simulink model "autopilot"  (R2016b)
settings: Solver=VariableStepAuto  StartTime=0.0  StopTime=sim_time  RelTol=1e-3
values from neighbouring files (symbols this model uses):
  d = 0    [run_task_2e.m]
  k_i_chi = omega_n_chi^2 * V_g / g    [prob2b.m]
  k_p_chi = 2 * zeta_chi * omega_n_chi * V_g / g    [prob2b.m]
undefined symbols (not defined in the file or in its folder): a_phi_1, a_phi_2, delta_a_max, g, k_d_phi, k_i_phi, k_p_phi, V_g
libraries: aerolibconvert2 x1
settings Model: Creator=Alexandra  LastModifiedBy=HenningWard

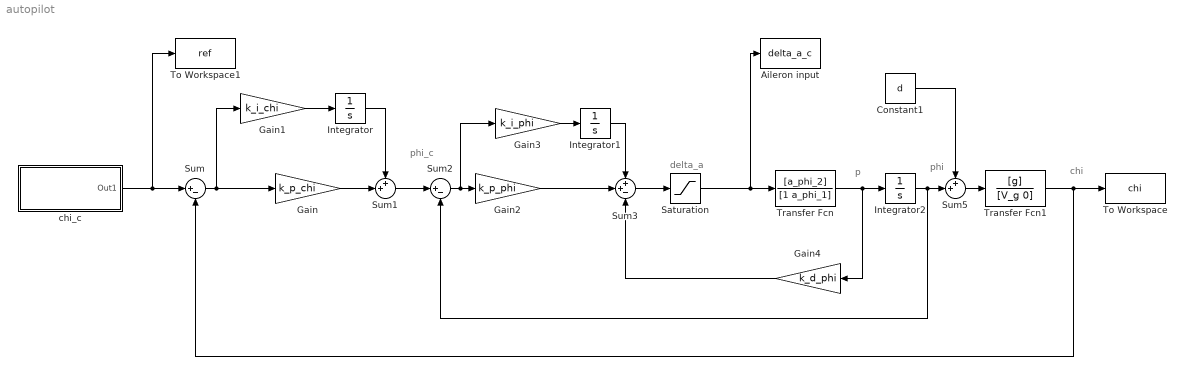
== system autopilot ==
  note: phi_c
  note: delta_a
  note: phi
  note: chi
  note: p
  Aileron input : ToWorkspace  VariableName=delta_a_c  SaveFormat=Structure With Time  SampleTime=-1
  Constant1 : Constant  Value=d
  Gain : Gain  Gain=k_p_chi
  Gain1 : Gain  Gain=k_i_chi
  Gain2 : Gain  Gain=k_p_phi
  Gain3 : Gain  Gain=k_i_phi
  Gain4 : Gain  Gain=k_d_phi
  Integrator : Integrator
  Integrator1 : Integrator
  Integrator2 : Integrator
  Saturation : Saturate  UpperLimit=delta_a_max  LowerLimit=-delta_a_max
  Sum : Sum  Inputs=|+-
  Sum1 : Sum  Inputs=++|
  Sum2 : Sum  Inputs=|+-
  Sum3 : Sum  Inputs=++-
  Sum5 : Sum  Inputs=++|
  To Workspace : ToWorkspace  VariableName=chi  SaveFormat=Structure With Time  SampleTime=-1
  To Workspace1 : ToWorkspace  VariableName=ref  SaveFormat=Structure With Time  SampleTime=-1
  Transfer Fcn : TransferFcn  Numerator=[a_phi_2]  Denominator=[1 a_phi_1]
  Transfer Fcn1 : TransferFcn  Numerator=[g]  Denominator=[V_g 0]
  chi_c : Subsystem
  wires:
  Sum/1 -> Gain1/1, Gain/1
  Gain1/1 -> Integrator/1
  Gain/1 -> Sum1/2
  Integrator/1 -> Sum1/1
  Sum1/1 -> Sum2/1
  Sum2/1 -> Gain3/1, Gain2/1
  Gain3/1 -> Integrator1/1
  Integrator1/1 -> Sum3/1
  Gain2/1 -> Sum3/2
  Transfer Fcn/1 -> Gain4/1, Integrator2/1
  Integrator2/1 -> Sum2/2, Sum5/2
  Gain4/1 -> Sum3/3
  Constant1/1 -> Sum5/1
  Sum5/1 -> Transfer Fcn1/1
  Transfer Fcn1/1 -> Sum/2, To Workspace/1
  Sum3/1 -> Saturation/1
  Saturation/1 -> Aileron input/1, Transfer Fcn/1
  chi_c/1(Out1) -> To Workspace1/1, Sum/1

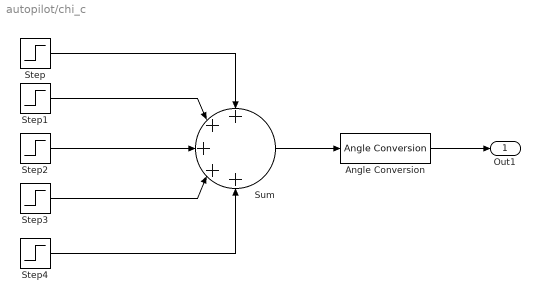
== system autopilot/chi_c ==
  Angle Conversion : aerolibconvert2/Angle Conversion  IU=deg  OU=rad
  Step : Step  Time=0  After=0  SampleTime=0
  Step1 : Step  Time=100  After=2  SampleTime=0
  Step2 : Step  Time=200  After=4  SampleTime=0
  Step3 : Step  Time=300  After=6  SampleTime=0
  Step4 : Step  Time=400  After=8  SampleTime=0
  Sum : Sum  Inputs=+++++
  Out1 : Outport
  wires:
  Step2/1 -> Sum/3
  Step1/1 -> Sum/2
  Step/1 -> Sum/1
  Step3/1 -> Sum/4
  Step4/1 -> Sum/5
  Sum/1 -> Angle Conversion/1
  Angle Conversion/1 -> Out1/1
